simulink model "untitled"  (Simulink 6.5)
settings: Solver=ode45  StartTime=0.0  StopTime=0.1  RelTol=1e-3
libraries: simulink_extras x1
settings Model: Creator=fl42597  LastModifiedBy=fl42597

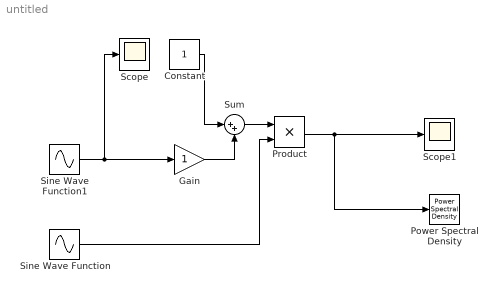
== system untitled ==
  Constant : Constant  Value=1  OutDataType=sfix(16)  ConRadixGroup=Use specified scaling  OutScaling=2^0  SampleTime=inf  FramePeriod=inf
  Gain : Gain
  Power Spectral Density : simulink_extras/Additional Sinks/Power Spectral Density  SystemSampleTime=-1  npts=1024  fftpts=2048  HowOften=512  sampleT=0.00001
  Product : Product  RndMeth=Zero
  Scope : Scope
  Scope1 : Scope
  Sine Wave Function : Sin  Frequency=5000*2*pi  SampleTime=0.00001
  Sine Wave Function1 : Sin  Frequency=500*2*pi  SampleTime=0.00001
  Sum : Sum  Inputs=|++
  wires:
  Sine Wave Function1/1 -> Gain/1, Scope/1
  Sine Wave Function/1 -> Product/2
  Product/1 -> Scope1/1, Power Spectral Density/1
  Gain/1 -> Sum/2
  Constant/1 -> Sum/1
  Sum/1 -> Product/1
